simulink library "SLDCMotors_Lib"  (R2014a)
settings: Solver=ode45  StartTime=0.0  StopTime=10.0  RelTol=1e-3
libraries: fl_lib x19, nesl_utility x8, SLDCMotors_Lib x1, cstblocks x1, elec_lib x1
settings Model: Creator=cosorio  LastModifiedBy=Sebastian

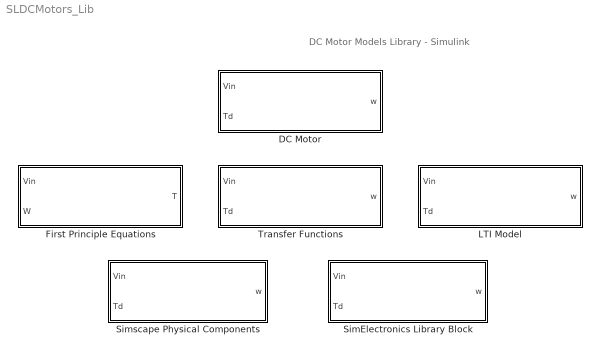
== system SLDCMotors_Lib ==
  note: DC Motor Models Library - Simulink
  DC Motor : Subsystem  BlockChoice=First Principle Equations
      settings: TemplateBlock=self  MemberBlocks=First Principle Equations,LTI Model,SimElectronics Library Block,Simscape Physical Components,Transfer Functions
  First Principle Equations : Subsystem  mask(DC Motor - First Principles){R=1, L=0.5, Kemf=0.1, Km=0.01}
      mask prompts: R "Armature Resistance (Ohms) :"; L "Armature Inductance (Henrys) :"; Kemf "Rotor Damping (N*m/(rad/s)) :"; Km "Torque/Back EMF Constant :"
  LTI Model : Subsystem  mask(DC Motor - LTI Model){R=1, L=0.5, Kf=0.1, J=0.01, Km=0.01}
      mask prompts: R "Armature Resistance (Ohms) :"; L "Armature Inductance (Henrys) :"; Kf "Rotor Damping (N*m/(rad/s)) :"; J "Rotor Inertia (kg*m^2) :"; Km "Torque/Back EMF Constant :"
      mask init:
      | Kemf = Km;
      | %%%%%
      | Gtorque = tf(Km,[L,R]);    
      | Gspeed = tf(1,[J,Kf]);
      | 
      | Gdc_motor = ss(Gspeed)*[Gtorque,1];
      | Gdc_motor = feedback(Gdc_motor,Kemf,1,1);
  SimElectronics Library Block : Subsystem  mask(DC Motor - SimElectronics Block){R=1, L=0.5, Kf=0.1, J=0.01, Km=0.01}
      mask prompts: R "Armature Resistance (Ohms) :"; L "Armature Inductance (Henrys) :"; Kf "Rotor Damping (N*m/(rad/s)) :"; J "Rotor Inertia (kg*m^2) :"; Km "Torque/Back EMF Constant"
  Simscape Physical Components : Subsystem  mask(DC Motor - Physical Components){R=1, L=0.5, Kf=0.1, J=0.01, Km=0.01}
      mask prompts: R "Armature Resistance (Ohms) :"; L "Armature Inductance (Henrys) :"; Kf "Rotor Damping (N*m/(rad/s)) :"; J "Rotor Inertia (kg*m^2) :"; Km "Torque/Back EMF Constant :"
  Transfer Functions : Subsystem  mask(DC Motor - Transfer Functions){R=1, L=0.5, Kf=0.1, J=0.01, Km=0.01}
      mask prompts: R "Armature Resistance (Ohms) :"; L "Armature Inductance (Henrys) :"; Kf "Rotor Damping (N*m/(rad/s)) :"; J "Rotor Inertia (kg*m^2) :"; Km "Torque/Back EMF Constant :"
      mask init:
      | Kemf = Km;

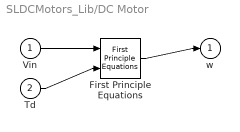
== system SLDCMotors_Lib/DC Motor ==
  Vin : Inport
  Td : Inport  Port=2
  First Principle Equations : SLDCMotors_Lib/First Principle Equations  R=1  L=0.5  Kemf=0.1  J=0.01  Km=0.01
  w : Outport
  wires:
  Vin/1 -> First Principle Equations/1
  Td/1 -> First Principle Equations/2
  First Principle Equations/1 -> w/1

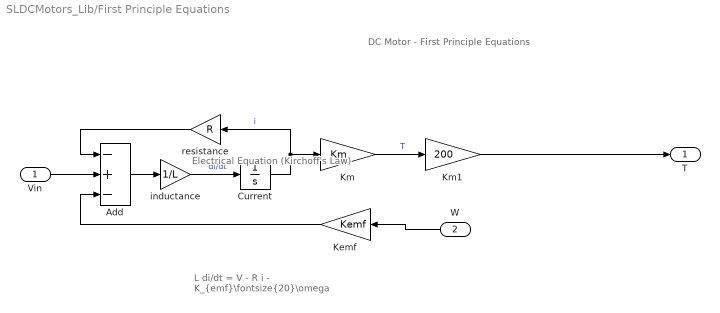
== system SLDCMotors_Lib/First Principle Equations ==
  note: L di/dt = V - R i - K_{emf}\fontsize{20}\omega
  note: DC Motor - First Principle Equations
  note: Electrical Equation
      | (Kirchoff's Law)
  Vin : Inport
  W : Inport  Port=2
  Add : Sum  Inputs=-+-
  Current : Integrator
  Kemf : Gain  Gain=Kemf
  Km : Gain  Gain=Km
  Km1 : Gain  Gain=200
  inductance : Gain  Gain=1/L
  resistance : Gain  Gain=R
  T : Outport
  wires:
  Vin/1 -> Add/2
  inductance/1 -> Current/1  "di/dt"
  Current/1 -> resistance/1, Km/1  "i"
  Add/1 -> inductance/1
  resistance/1 -> Add/1
  Kemf/1 -> Add/3
  W/1 -> Kemf/1
  Km/1 -> Km1/1  "T"
  Km1/1 -> T/1

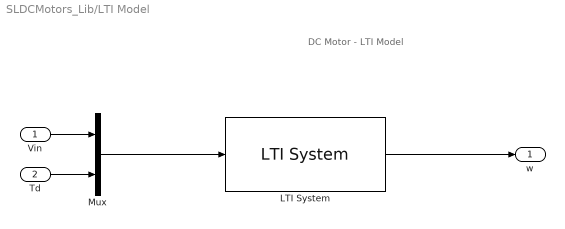
== system SLDCMotors_Lib/LTI Model ==
  note: DC Motor - LTI Model
  Vin : Inport
  Td : Inport  Port=2
  LTI System : cstblocks/LTI System  sys=Gdc_motor  IC=[]
  Mux : Mux  Inputs=2
  w : Outport
  wires:
  LTI System/1 -> w/1
  Mux/1 -> LTI System/1
  Vin/1 -> Mux/1
  Td/1 -> Mux/2

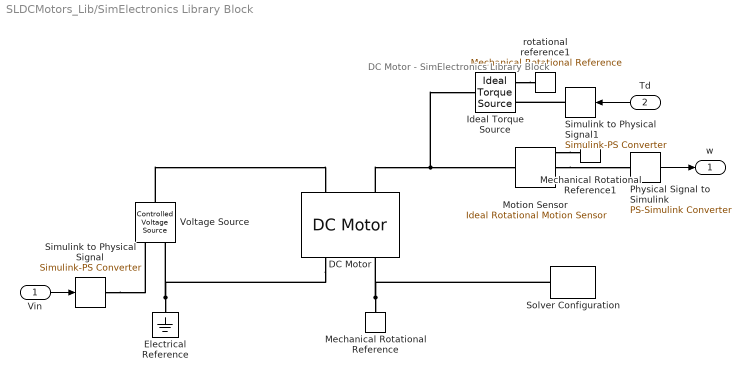
== system SLDCMotors_Lib/SimElectronics Library Block ==
  note: DC Motor - SimElectronics Library Block
  Vin : Inport
  Td : Inport  Port=2
  DC Motor : elec_lib/Actuators & Drivers/Rotational Actuators/DC Motor  parameterization=1  Ra=R Ohm  La=L H  emf_or_torque=2  Kv=7.2e-05 V/rpm  Ki=Km N*m/A  T_stall=2.4e-04 N*m  w_max=1.91e+04 rpm  w_rated=1.5e+04 rpm  P_rated=0.08 W  V_rated=1.5 V  J=J kg*m^2  lam_param=1  lam=Kf N*m/(rad/s)  i_noload=0 A  V_i_noload=1.5 V  speed0=0 rpm  alpha=0.00393 1/K  Tmeas=25 C  thermal_mass=100 J/K  initial_temperature=25 C
  Electrical Reference : fl_lib/Electrical/Electrical Elements/Electrical Reference
  Ideal Torque Source : fl_lib/Mechanical/Mechanical Sources/Ideal Torque Source
  Mechanical Rotational Reference : fl_lib/Mechanical/Rotational Elements/Mechanical Rotational Reference
  Mechanical Rotational Reference1 : fl_lib/Mechanical/Rotational Elements/Mechanical Rotational Reference
  Motion Sensor : fl_lib/Mechanical/Mechanical Sensors/Ideal Rotational Motion Sensor  offset=0 rad
  Physical Signal to Simulink : nesl_utility/PS-Simulink Converter  PhysicalDomain=network_engine_domain  SubClassName=ps_output  LeftPortType=input  RightPortType=output  PseudoPeriodic=off  Frequencies=[]  Unit=rad/s  AffineConversion=off
  Simulink to Physical Signal : nesl_utility/Simulink-PS Converter  PhysicalDomain=network_engine_domain  SubClassName=ps_input  LeftPortType=input  RightPortType=output  PseudoPeriodic=off  Frequencies=[]  NoiseDistribution=none  NoiseParameters=[]  Unit=V  AffineConversion=off  InputFiltering=off  SimscapeFilterOrder=1  InputFilterTimeConstant=.001  UdotUserProvided=0
  Simulink to Physical Signal1 : nesl_utility/Simulink-PS Converter  PhysicalDomain=network_engine_domain  SubClassName=ps_input  LeftPortType=input  RightPortType=output  PseudoPeriodic=off  Frequencies=[]  NoiseDistribution=none  NoiseParameters=[]  Unit=1  AffineConversion=off  InputFiltering=off  SimscapeFilterOrder=1  InputFilterTimeConstant=.001  UdotUserProvided=0
  Solver Configuration : nesl_utility/Solver Configuration  PhysicalDomain=network_engine_domain  SubClassName=solver  LeftPortType=input  RightPortType=generic  Accelerate=off  Tones=[]  Harmonics=[]  SimulateNoise=off  Profile=off  UseLocalSampling=off  EnableSwitchedLinearOptims=on  FrequencyDomain=off  UseCCode=off  RelTol=0.001  AbsTol=1e-06  MinStep=1e-09  ToWorkspace=off  DoDC=off  ResidualTolerance=1e-9  UseLocalSolver=off  LocalSolverChoice=NE_BACKWARD_EULER_ADVANCER  LocalSolverSampleTime=.001  DoFixedCost=off  MaxNonlinIter=12  MaxModeIter=2  LinearAlgebra=Sparse  DelaysMemoryBudget=1024  AutomaticFiltering=on  FilteringTimeConstant=0.001
  Voltage Source : fl_lib/Electrical/Electrical Sources/Controlled Voltage Source
  rotational reference1 : fl_lib/Mechanical/Rotational Elements/Mechanical Rotational Reference
  w : Outport
  wires:
  Physical Signal to Simulink/1 -> w/1
  Vin/1 -> Simulink to Physical Signal/1
  Td/1 -> Simulink to Physical Signal1/1
  connections:
  Motion Sensor/RConn1 -- Mechanical Rotational Reference1/LConn1
  Mechanical Rotational Reference/LConn1 -- DC Motor/RConn2 -- Solver Configuration/RConn1
  DC Motor/LConn2 -- Motion Sensor/LConn1 -- Ideal Torque Source/LConn1
  Motion Sensor/RConn2 -- Physical Signal to Simulink/LConn1
  Electrical Reference/LConn1 -- Voltage Source/RConn2 -- DC Motor/RConn1
  Voltage Source/LConn1 -- DC Motor/LConn1
  Simulink to Physical Signal/RConn1 -- Voltage Source/RConn1
  Simulink to Physical Signal1/RConn1 -- Ideal Torque Source/RConn1
  Ideal Torque Source/RConn2 -- rotational reference1/LConn1

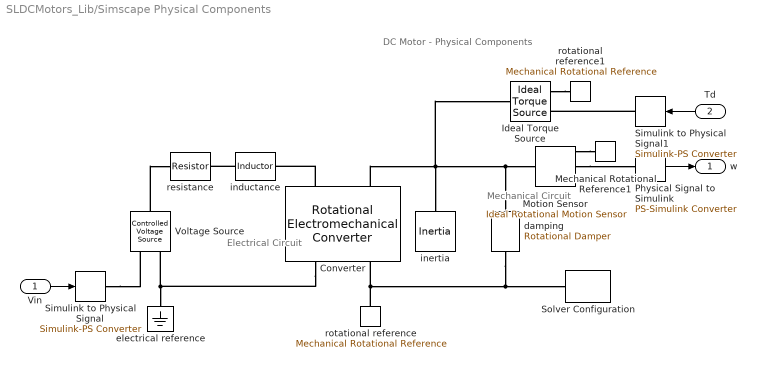
== system SLDCMotors_Lib/Simscape Physical Components ==
  note: Mechanical Circuit
  note: Electrical Circuit
  note: DC Motor - Physical Components
  Vin : Inport
  Td : Inport  Port=2
  Converter : fl_lib/Electrical/Electrical Elements/Rotational Electromechanical Converter  K=Km V/(rad/s)  i_specify=off  i_priority=High  i=0 A  v_specify=off  v_priority=High  v=0 V  t_specify=off  t_priority=High  t=0 N*m  w_specify=off  w_priority=High  w=0 rad/s
  Ideal Torque Source : fl_lib/Mechanical/Mechanical Sources/Ideal Torque Source
  Mechanical Rotational Reference1 : fl_lib/Mechanical/Rotational Elements/Mechanical Rotational Reference
  Motion Sensor : fl_lib/Mechanical/Mechanical Sensors/Ideal Rotational Motion Sensor  offset=0 rad
  Physical Signal to Simulink : nesl_utility/PS-Simulink Converter  PhysicalDomain=network_engine_domain  SubClassName=ps_output  LeftPortType=input  RightPortType=output  PseudoPeriodic=off  Frequencies=[]  Unit=rad/s  AffineConversion=off
  Simulink to Physical Signal : nesl_utility/Simulink-PS Converter  PhysicalDomain=network_engine_domain  SubClassName=ps_input  LeftPortType=input  RightPortType=output  PseudoPeriodic=off  Frequencies=[]  NoiseDistribution=none  NoiseParameters=[]  Unit=V  AffineConversion=off  InputFiltering=off  SimscapeFilterOrder=1  InputFilterTimeConstant=.001  UdotUserProvided=0
  Simulink to Physical Signal1 : nesl_utility/Simulink-PS Converter  PhysicalDomain=network_engine_domain  SubClassName=ps_input  LeftPortType=input  RightPortType=output  PseudoPeriodic=off  Frequencies=[]  NoiseDistribution=none  NoiseParameters=[]  Unit=1  AffineConversion=off  InputFiltering=off  SimscapeFilterOrder=1  InputFilterTimeConstant=.001  UdotUserProvided=0
  Solver Configuration : nesl_utility/Solver Configuration  PhysicalDomain=network_engine_domain  SubClassName=solver  LeftPortType=input  RightPortType=generic  Accelerate=off  Tones=[]  Harmonics=[]  SimulateNoise=off  Profile=off  UseLocalSampling=off  EnableSwitchedLinearOptims=on  FrequencyDomain=off  UseCCode=off  RelTol=0.001  AbsTol=1e-06  MinStep=1e-09  ToWorkspace=off  DoDC=off  ResidualTolerance=1e-9  UseLocalSolver=off  LocalSolverChoice=NE_BACKWARD_EULER_ADVANCER  LocalSolverSampleTime=.001  DoFixedCost=off  MaxNonlinIter=12  MaxModeIter=2  LinearAlgebra=Sparse  DelaysMemoryBudget=1024  AutomaticFiltering=on  FilteringTimeConstant=0.001
  Voltage Source : fl_lib/Electrical/Electrical Sources/Controlled Voltage Source
  damping : fl_lib/Mechanical/Rotational Elements/Rotational Damper  D=Kf N*m/(rad/s)  w_specify=off  w_priority=High  w=0 rad/s  t_specify=off  t_priority=High  t=0 N*m
  electrical reference : fl_lib/Electrical/Electrical Elements/Electrical Reference
  inductance : fl_lib/Electrical/Electrical Elements/Inductor  l=L H  r=0 Ohm  g=1e-09 1/Ohm  i_specify=off  i_priority=High  i=0 A  v_specify=off  v_priority=High  v=0 V  i_L_specify=on  i_L_priority=High  i_L=0 A
  inertia : fl_lib/Mechanical/Rotational Elements/Inertia  inertia=J kg*m^2  w_specify=on  w_priority=High  w=0 rad/s  t_specify=off  t_priority=High  t=0 N*m
  resistance : fl_lib/Electrical/Electrical Elements/Resistor  Tag=Factory Generic  R=R Ohm  i_specify=off  i_priority=High  i=0 A  v_specify=off  v_priority=High  v=0 V
  rotational reference : fl_lib/Mechanical/Rotational Elements/Mechanical Rotational Reference
  rotational reference1 : fl_lib/Mechanical/Rotational Elements/Mechanical Rotational Reference
  w : Outport
  wires:
  Physical Signal to Simulink/1 -> w/1
  Vin/1 -> Simulink to Physical Signal/1
  Td/1 -> Simulink to Physical Signal1/1
  connections:
  Motion Sensor/RConn1 -- Mechanical Rotational Reference1/LConn1
  Motion Sensor/RConn2 -- Physical Signal to Simulink/LConn1
  damping/LConn1 -- Motion Sensor/LConn1 -- inertia/LConn1 -- Converter/LConn2 -- Ideal Torque Source/LConn1
  inductance/LConn1 -- resistance/RConn1
  Converter/LConn1 -- inductance/RConn1
  damping/RConn1 -- Solver Configuration/RConn1 -- Converter/RConn2 -- rotational reference/LConn1
  Converter/RConn1 -- electrical reference/LConn1 -- Voltage Source/RConn2
  Voltage Source/LConn1 -- resistance/LConn1
  Simulink to Physical Signal/RConn1 -- Voltage Source/RConn1
  Simulink to Physical Signal1/RConn1 -- Ideal Torque Source/RConn1
  Ideal Torque Source/RConn2 -- rotational reference1/LConn1

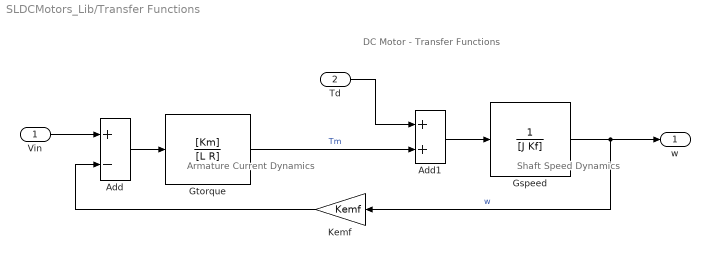
== system SLDCMotors_Lib/Transfer Functions ==
  note: Armature Current Dynamics
  note: DC Motor - Transfer Functions
  note: Shaft Speed Dynamics
  Vin : Inport
  Td : Inport  Port=2
  Add : Sum  Inputs=+-
  Add1 : Sum
  Gspeed : TransferFcn  Denominator=[J Kf]
  Gtorque : TransferFcn  Numerator=[Km]  Denominator=[L R]
  Kemf : Gain  Gain=Kemf
  w : Outport
  wires:
  Add/1 -> Gtorque/1
  Add1/1 -> Gspeed/1
  Gspeed/1 -> w/1, Kemf/1  "w"
  Vin/1 -> Add/1
  Td/1 -> Add1/1
  Gtorque/1 -> Add1/2  "Tm"
  Kemf/1 -> Add/2
